simulink model "condenser2020b"  (R2020b)
settings: Solver=VariableStepAuto  StartTime=0.0  StopTime=10.0  RelTol=1e-3
settings Model: Creator=Adam  LastModifiedBy=Adam

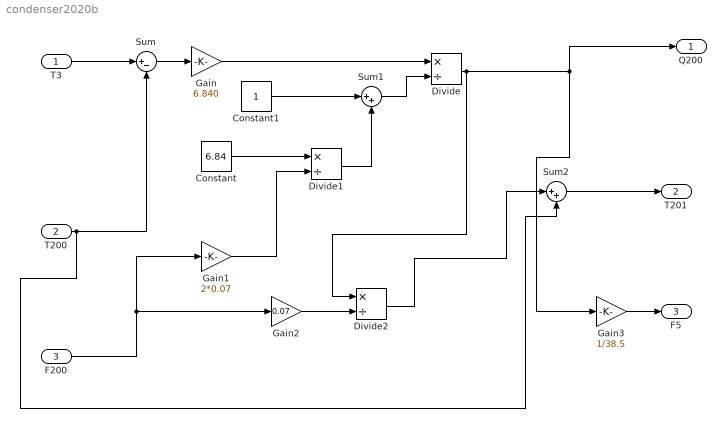
== system condenser2020b ==
  T3 : Inport
  T200 : Inport  Port=2
  F200 : Inport  Port=3
  Constant : Constant  Value=6.84
  Constant1 : Constant
  Divide : Product  Inputs=*/
  Divide1 : Product  Inputs=*/
  Divide2 : Product  Inputs=*/
  Gain : Gain  Gain=6.840
  Gain1 : Gain  Gain=2*0.07
  Gain2 : Gain  Gain=0.07
  Gain3 : Gain  Gain=1/38.5
  Sum : Sum  Inputs=|+-
  Sum1 : Sum  Inputs=|++
  Sum2 : Sum  Inputs=|++
  Q200 : Outport
  T201 : Outport  Port=2
  F5 : Outport  Port=3
  wires:
  T200/1 -> Sum/2, Sum2/2
  T3/1 -> Sum/1
  Sum/1 -> Gain/1
  Gain/1 -> Divide/1
  F200/1 -> Gain2/1, Gain1/1
  Constant/1 -> Divide1/1
  Gain1/1 -> Divide1/2
  Sum1/1 -> Divide/2
  Constant1/1 -> Sum1/1
  Divide1/1 -> Sum1/2
  Divide/1 -> Divide2/1, Gain3/1, Q200/1
  Gain2/1 -> Divide2/2
  Divide2/1 -> Sum2/1
  Sum2/1 -> T201/1
  Gain3/1 -> F5/1
